simulink model "MIMOSystemAntenna"  (R2021a)
settings: Solver=FixedStepDiscrete  StartTime=0.0  StopTime=inf  RelTol=1e-3
PreLoadFcn:
  | Sig_Ang=120;
  | Int_Ang=90;
  | Frame = 32;
  | load dipoleArray;
InitFcn:
  | load dipoleArray;
values from neighbouring files (symbols this model uses):
  F0 = 5000000000    [dipoleArray.mat]
  L = [9.00164081673e-10 1.08900441217e-09 1.17350873052e-09 1.12597709024e-09 1.12597709023e-09 1.17350873052e-09 1.08900441217e-09 9.00164081661e-10]    [dipoleArray.mat]
  lambda = 0.0599584916    [dipoleArray.mat]
undefined symbols (not defined in the file or in its folder): comm, constellation, design, dipole, if_filt, magnitude, pattern, phased, physconst, rf_filt, S
libraries: simrfV2elements x41, simrfV2util1 x17, simulink_extras x16, simrfV2systems x8, simrfV2sources1 x8, commfilt2 x2, dspmathops x2, commrflib2 x1, dspsrcs4 x1, phasedbflib x1, phaseddoalib x1, commrfcorlib x1
settings Model: SimulationMode=accelerator  NumberOfSteps=8  Creator=shmueld  LastModifiedBy=Michael
settings SolverCC: AlgebraicLoopSolver=TrustRegion  MinimalZcImpactIntegration=on
settings DataIOCC: SaveFormat=Array  SaveOutput=off  SignalLogging=off  DSMLogging=off  VisualizeSimOutput=off  SaveTime=off  ReturnWorkspaceOutputs=off
settings OptimizationCC: DefaultParameterBehavior=Inlined  InlineInvariantSignals=on  EfficientMapNaN2IntZero=off  LifeSpan=inf
settings DebuggingCC: RTPrefix=none  ReadBeforeWriteMsg=DisableAll  WriteAfterWriteMsg=DisableAll  WriteAfterReadMsg=DisableAll  AlgebraicLoopMsg=none  ArtificialAlgebraicLoopMsg=none  MaxConsecutiveZCsMsg=none  InheritedTsInSrcMsg=none  MultiTaskDSMMsg=none  MultiTaskCondExecSysMsg=none  MultiTaskRateTransMsg=warning  TasksWithSamePriorityMsg=none  SigSpecEnsureSampleTimeMsg=none  IntegerOverflowMsg=none  Int32ToFloatConvMsg=none  ParameterDowncastMsg=none  ParameterOverflowMsg=none  ParameterPrecisionLossMsg=none  ParameterTunabilityLossMsg=none  FcnCallInpInsideContextMsg=warning  UnconnectedInputMsg=none  UnconnectedOutputMsg=none  UnconnectedLineMsg=none  FrameProcessingCompatibilityMsg=none  BusObjectLabelMismatch=none  RootOutportRequireBusObject=none  AllowSymbolicDim=off  UnknownTsInhSupMsg=none  ModelReferenceDataLoggingMessage=none  ModelReferenceExtraNoncontSigs=none  OperatingPointInterfaceChecksumMismatchMsg=none  NonCurrentReleaseOperatingPointMsg=warning  PregeneratedLibrarySubsystemCodeDiagnostic=none  SFUnusedDataAndEventsDiag=none  SFUnexpectedBacktrackingDiag=none  SFInvalidInputDataAccessInChartInitDiag=none  SFNoUnconditionalDefaultTransitionDiag=none  SFTransitionOutsideNaturalParentDiag=none  SFUnreachableExecutionPathDiag=none  SFUndirectedBroadcastEventsDiag=none  SFTransitionActionBeforeConditionDiag=none  SFOutputUsedAsStateInMooreChartDiag=none  SFExecutionAtInitializationDiag=none  SFMachineParentedDataDiag=warning  IntegerSaturationMsg=none  ArithmeticOperatorsInVariantConditions=warning
settings HardwareCC: ProdBitPerPointer=32  ProdBitPerSizeT=32  ProdBitPerPtrDiffT=32  ProdLargestAtomicFloat=None  ProdIntDivRoundTo=Undefined  ProdEndianess=Unspecified  ProdWordSize=32  ProdHWDeviceType=32-bit Generic  TargetBitPerPointer=64  TargetBitPerSizeT=64  TargetBitPerPtrDiffT=64  TargetLongLongMode=on  TargetIntDivRoundTo=Zero  TargetEndianess=LittleEndian  TargetWordSize=64  TargetHWDeviceType=MATLAB Host  ProdEqTarget=off
settings ModelReferenceCC: UpdateModelReferenceTargets=IfOutOfDate  PropagateSignalLabelsOutOfModel=off
settings SFSimCC: SFSimEcho=off  SimUseLocalCustomCode=off  CustomCodeUndefinedFunction=UseInterfaceOnly
settings RTWCC: RTWUseLocalCustomCode=off
settings CodeAppCC: MaxIdLength=128
settings GRTTargetCC: TargetLangStandard=C89/C90 (ANSI)  CombineOutputUpdateFcns=off  GRTInterface=on
settings ConfigComp: CovMetricSettings=dw  CovSaveCumulativeToWorkspaceVar=on  CovSaveSingleToWorkspaceVar=on  CovExternalEMLEnable=off
settings SimscapeCC: ExplicitSolverDiagnosticOptions=none  SimscapeNormalizeSystem=off

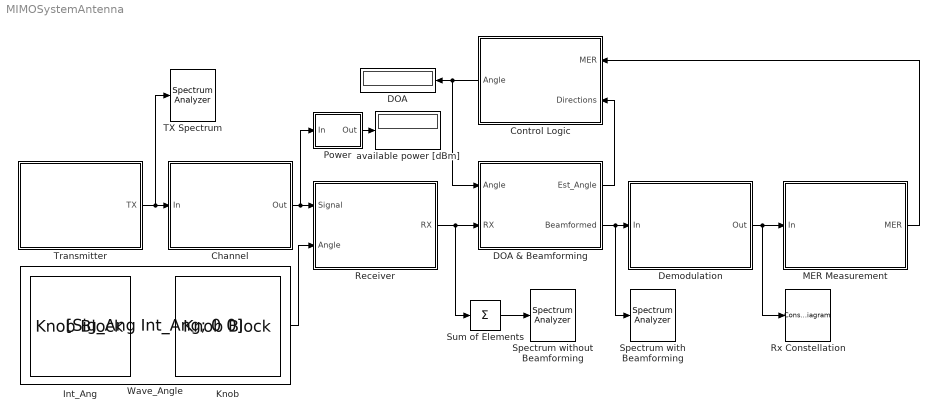
== system MIMOSystemAntenna ==
  Channel : Subsystem  mask{PathLoss=60, PowInterf=-20}
      mask prompts: PathLoss "Path loss (dB)"; PowInterf "Interfering signal power (dBm)"
  Control Logic : Subsystem
  DOA : Display
  DOA & Beamforming : Subsystem
  Demodulation : Subsystem
  Int_Ang : KnobBlock  ScaleMax=180  TickInterval=30
  Knob : KnobBlock  ScaleMax=180  TickInterval=30
  MER Measurement : Subsystem
  "Power  " : Subsystem  mask{R=1}
      mask prompts: R "Reference Impedance [Ohm]"
      mask DialogControl DescGroupVar Prompt: Power Meter
  Receiver : Subsystem
  Rx Constellation : ConstellationDiagram
  Spectrum with Beamforming : SpectrumAnalyzer
  Spectrum without Beamforming : SpectrumAnalyzer
  Sum of Elements : Sum  Inputs=+
  TX Spectrum : SpectrumAnalyzer
  Transmitter : Subsystem
  Wave_Angle : Constant  Value=[Sig_Ang Int_Ang; 0 0]  VectorParams1D=off
      mask Display: disp('')
  available power [dBm] : Display
  wires:
  DOA & Beamforming/2(Beamformed) -> Demodulation/1(In), Spectrum with Beamforming/1
  Sum of Elements/1 -> Spectrum without Beamforming/1
  Transmitter/1(TX) -> TX Spectrum/1, Channel/1(In)
  Receiver/1(RX) -> Sum of Elements/1, DOA & Beamforming/2(RX)
  Channel/1(Out) -> "Power  "/1(In), Receiver/1(Signal)
  Wave_Angle/1 -> Receiver/2(Angle)
  Control Logic/1(Angle) -> DOA & Beamforming/1(Angle), DOA/1
  MER Measurement/1(MER) -> Control Logic/1(MER)
  DOA & Beamforming/1(Est_Angle) -> Control Logic/2(Directions)
  Demodulation/1(Out) -> MER Measurement/1(In), Rx Constellation/1
  "Power  "/1(Out) -> available power [dBm]/1

== system MIMOSystemAntenna/Channel ==
  In : Inport
  Free Space Path Loss1 : commrflib2/Free Space Path Loss  mode=Decibels  dB=PathLoss  d=0.100  fc=1920
      settings: SourceProductBaseCode=CM
  Interferer : dspsrcs4/Sine Wave  Amplitude=10^((PowInterf-30)/20)  Frequency=2.5e6  Phase=0  SampleMode=Discrete  OutComplex=Complex  CompMethod=Trigonometric fcn  TableSize=Speed  SampleTime=8.6806e-8  SamplesPerFrame=1  ResetState=Restart at time zero  OutputFrames=off  dataType=double  wordLen=16  udDataType=sfix(16)  fracBitsMode=Best precision  numFracBits=15  OutDataTypeStr=double  LastOutDataTypeStr=double
  Vector Concatenate1 : Concatenate  Mode=Multidimensional array  ConcatenateDimension=2
  Out : Outport  VectorParamsAs1DForOutWhenUnconnected=off
  wires:
  Free Space Path Loss1/1 -> Vector Concatenate1/1  "Input RX"
  Vector Concatenate1/1 -> Out/1
  In/1 -> Free Space Path Loss1/1
  Interferer/1 -> Vector Concatenate1/2

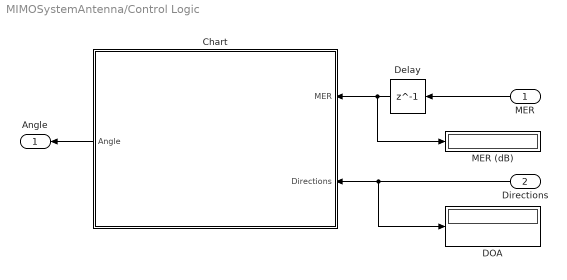
== system MIMOSystemAntenna/Control Logic ==
  MER : Inport
  Directions : Inport  Port=2
  Chart : Stateflow chart  TreatAsAtomicUnit=on
  DOA : Display
  Delay : Delay  DelayLength=1  InitialCondition=0
  MER (dB) : Display
  Angle : Outport  VectorParamsAs1DForOutWhenUnconnected=off
  wires:
  Delay/1 -> Chart/1(MER), MER (dB)/1
  Directions/1 -> Chart/2(Directions), DOA/1
  Chart/1(Angle) -> Angle/1
  MER/1 -> Delay/1

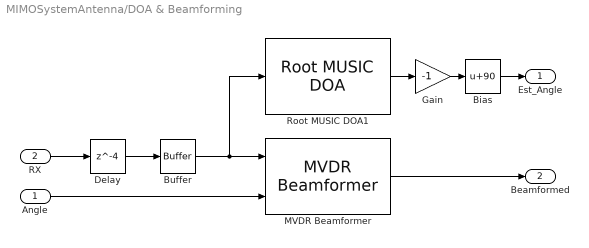
== system MIMOSystemAntenna/DOA & Beamforming ==
  Angle : Inport
  RX : Inport  Port=2
  Bias : Bias  Bias=90
  Buffer : Buffer  N=Frame  OutputFrames=off
  Delay : Delay  DelayLength=4  InitialCondition=1
  Gain : Gain  Gain=-1
  MVDR Beamformer : phasedbflib/MVDR Beamformer  PropagationSpeed=physconst( 'LightSpeed' )  OperatingFrequency=F0  DiagonalLoadingFactor=0.1  TrainingInputPort=off  DirectionSource=Input port  Direction=[ 0; 0 ]  NumPhaseShifterBits=0  WeightsOutputPort=off  SimulateUsing=Interpreted execution  SensorArray=phased.ULA('Element',phased.CustomAntennaElement('AzimuthAngles',-180:5:180,'ElevationAngles',-90:5:90,'MagnitudePattern',pattern(design(dipole,F0), F0),'PhasePattern',zeros(37,73)),'NumElements',8,'ElementSpacing',0.5*lambda,'ArrayAxis','x')
      settings: SourceProductBaseCode=AR
  Root MUSIC DOA1 : phaseddoalib/Root MUSIC DOA  PropagationSpeed=physconst( 'LightSpeed' )  OperatingFrequency=F0  NumSignalsSource=Property  NumSignalsMethod=AIC  NumSignals=2  ForwardBackwardAveraging=on  SpatialSmoothing=0  SimulateUsing=Interpreted execution  SensorArray=phased.ULA('Element',phased.CustomAntennaElement('AzimuthAngles',-180:5:180,'ElevationAngles',-90:5:90,'MagnitudePattern',pattern(design(dipole,F0), F0),'PhasePattern',zeros(37,73)),'NumElements',8,'ArrayAxis','x','ElementSpacing',0.5*lambda)
      settings: SourceProductBaseCode=AR
  Est_Angle : Outport  VectorParamsAs1DForOutWhenUnconnected=off
  Beamformed : Outport  Port=2  VectorParamsAs1DForOutWhenUnconnected=off
  wires:
  Gain/1 -> Bias/1
  Bias/1 -> Est_Angle/1
  RX/1 -> Delay/1
  Root MUSIC DOA1/1 -> Gain/1
  Buffer/1 -> MVDR Beamformer/1, Root MUSIC DOA1/1
  MVDR Beamformer/1 -> Beamformed/1
  Delay/1 -> Buffer/1
  Angle/1 -> MVDR Beamformer/2

== system MIMOSystemAntenna/Demodulation ==
  In : Inport
  AGC : commrfcorlib/AGC  LegacyMode=off  DetectorMethod=Rectifier  LoopMethod=Linear  UpdatePeriod=100  StepSize=0.1  AdaptationStepSize=0.01  DesiredOutputPower=1/8  AveragingLength=64  MaximumGain=30  MaxPowerGain=60  GainOutputPort=off  InputPowerOutputPort=off  SimulateUsing=Interpreted execution
  Raised Cosine Receive Filter : commfilt2/Raised Cosine Receive Filter  filtType=Square root  R=0.2  filtSpan=8  N=8  downFactor=8  downOffset=0  filterGain=1  InputProcessing=Columns as channels (frame based)  RateOptions=Enforce single-rate processing  framing=Mute  checkCoeff=off  variableName=rcRxFilt  currentFiltSpan=8  D=(8)/2  inputOffset=0  sampMode=Mute  saveAsFlag=0  rateMode=Downsampling  checkGain=Normalized  launchFVT=on  roundingMode=Floor  overflowMode=off  coeffDataTypeStr=Inherit: Same word length as input  coeffMin=[]  coeffMax=[]  coeffLastDataTypeStr=Inherit: Same word length as input  accumDataTypeStr=Inherit: Same as product output  accumLastDataTypeStr=Inherit: Same as product output  outputDataTypeStr=Inherit: Same as accumulator  outputMin=[]  outputMax=[]  outputLastDataTypeStr=Inherit: Same as accumulator
  Out : Outport  VectorParamsAs1DForOutWhenUnconnected=off
      settings: SignalType=complex
  wires:
  AGC/1 -> Raised Cosine Receive Filter/1
  In/1 -> AGC/1
  Raised Cosine Receive Filter/1 -> Out/1

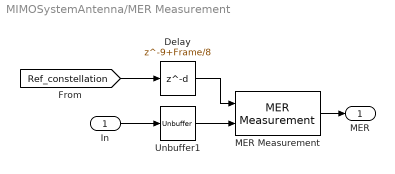
== system MIMOSystemAntenna/MER Measurement ==
  In : Inport
  Delay : Delay  DelayLength=9+Frame/8
  MER Measurement : commutil2/MER Measurement  ReferenceSignalSource=Input port  ReferenceConstellation=constellation( comm.QPSKModulator )  MeasurementIntervalSource=Custom  MeasurementInterval=8  AveragingDimensions=1  MinimumMEROutputPort=off  XPercentileMEROutputPort=off  XPercentileValue=95  SymbolCountOutputPort=off  SimulateUsing=Interpreted execution
      settings: SourceProductBaseCode=CM
  Unbuffer1 : Unbuffer
  MER : Outport  VectorParamsAs1DForOutWhenUnconnected=off
  wires:
  MER Measurement/1 -> MER/1
  Delay/1 -> MER Measurement/1
  [Ref_constellation] -> Delay/1
  In/1 -> Unbuffer1/1
  Unbuffer1/1 -> MER Measurement/2

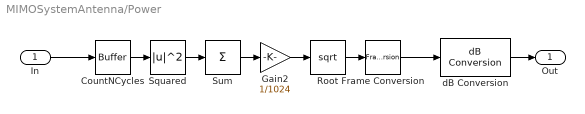
== system MIMOSystemAntenna/Power   ==
  In : Inport
  CountNCycles : Buffer  N=1024
  Frame Conversion : FrameConversion  OutFrame=Sample-based
  Gain2 : Gain  Gain=1/1024
  Root : Sqrt  SaturateOnIntegerOverflow=on
  Squared : Math  Operator=magnitude^2  SignedPower=on  SaturateOnIntegerOverflow=on
  Sum : Sum  Inputs=+  CollapseMode=Specified dimension
  dB Conversion : dspmathops/dB Conversion  dBtype=dBm  intype=Amplitude  R=R  fuzz=on
  Out : Outport  VectorParamsAs1DForOutWhenUnconnected=off
  wires:
  dB Conversion/1 -> Out/1
  In/1 -> CountNCycles/1
  Frame Conversion/1 -> dB Conversion/1
  CountNCycles/1 -> Squared/1
  Squared/1 -> Sum/1
  Sum/1 -> Gain2/1
  Root/1 -> Frame Conversion/1
  Gain2/1 -> Root/1

== system MIMOSystemAntenna/Receiver ==
  Signal : Inport
  Angle : Inport  Port=2
  Narrowband_Receive_Array : phasedtxrxlib/Narrowband Receive Array  PropagationSpeed=physconst( 'LightSpeed' )  OperatingFrequency=F0  Wavefront=Plane  SensorGainMeasure=dB  Polarization=None  WeightsInputPort=off  SimulateUsing=Interpreted execution  Sensor=phased.ULA('Element',phased.CustomAntennaElement('AzimuthAngles',-180:5:180,'ElevationAngles',-90:5:90,'MagnitudePattern',pattern(design(dipole,F0), F0),'PhasePattern',zeros(37,73)),'NumElements',8,'ElementSpacing',0.5*lambda,'ArrayAxis','x')
      settings: SourceProductBaseCode=AR
  RF_Receiver : Subsystem
  RX : Outport  VectorParamsAs1DForOutWhenUnconnected=off
  wires:
  Angle/1 -> Narrowband_Receive_Array/2
  Signal/1 -> Narrowband_Receive_Array/1
  Narrowband_Receive_Array/1 -> RF_Receiver/1(In)
  RF_Receiver/1(Out) -> RX/1

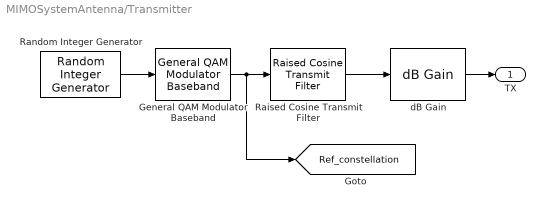
== system MIMOSystemAntenna/Transmitter ==
  General QAM Modulator Baseband : commdigbbndam3/General QAM Modulator Baseband  SigCon=[exp(2*pi*1i*[0:7]/8)]  outDtype=double  outWordLen=16  outUDDataType=sfix(16)  outFracLenMode=Best precision  outFracLen=15  outDataTypeStr=double  outLastDataTypeStr=double
      settings: SourceProductBaseCode=CM
  Raised Cosine Transmit Filter : commfilt2/Raised Cosine Transmit Filter  filtType=Square root  R=0.2  filtSpan=8  N=8  filterGain=1  InputProcessing=Columns as channels (frame based)  RateOptions=Allow multirate processing  framing=Mute  checkCoeff=off  variableName=rcTxFilt  checkGain=Normalized  sampMode=Mute  saveAsFlag=0  currentFiltSpan=8  D=(8)/2  launchFVT=on  roundingMode=Floor  overflowMode=off  coeffDataTypeStr=Inherit: Same word length as input  coeffMin=[]  coeffMax=[]  coeffLastDataTypeStr=Inherit: Same word length as input  outputDataTypeStr=Inherit: Same as accumulator  outputMin=[]  outputMax=[]  outputLastDataTypeStr=Inherit: Same as accumulator
  Random Integer Generator : commrandsrc3/Random Integer Generator  SetSize=8  SeedSource=Parameter  Seed=123456  SampleTime=8.6806e-8*8  SamplesPerFrame=1  OutputDataType=double  SimulateUsing=Interpreted execution
  dB Gain : dspmathops/dB Gain  dB=20  intype=Amplitude
      settings: SourceProductBaseCode=DS
  TX : Outport  VectorParamsAs1DForOutWhenUnconnected=off
  tag scope: Ref_constellation=global
  wires:
  Raised Cosine Transmit Filter/1 -> dB Gain/1
  General QAM Modulator Baseband/1 -> [Ref_constellation], Raised Cosine Transmit Filter/1
  Random Integer Generator/1 -> General QAM Modulator Baseband/1
  dB Gain/1 -> TX/1

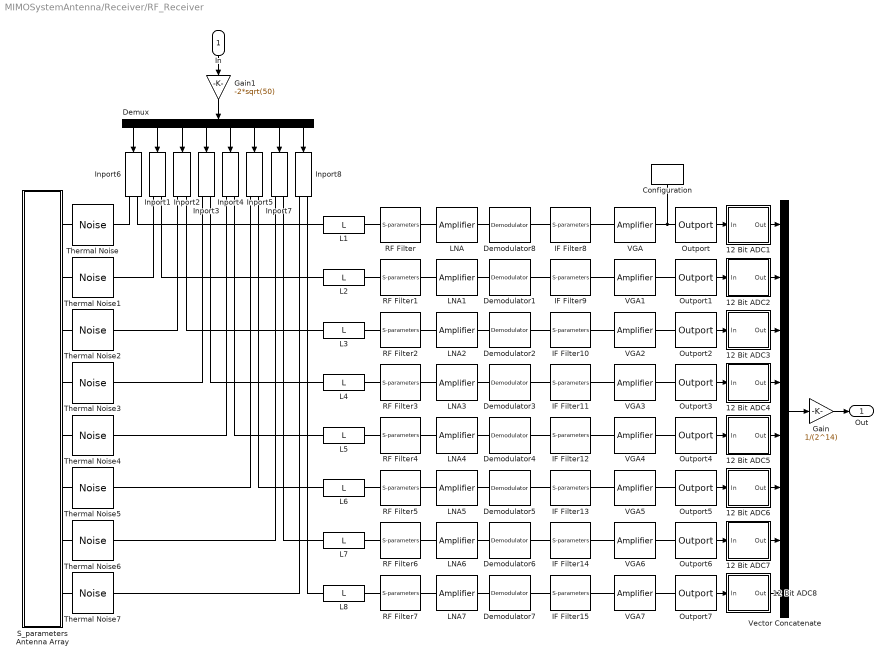
== system MIMOSystemAntenna/Receiver/RF_Receiver ==
  In : Inport
  12 Bit ADC1 : Subsystem  mask{FS_P_dBm=18, N=12}
      mask prompts: FS_P_dBm "Full Scale Power (dBm)"
  12 Bit ADC2 : Subsystem  mask{FS_P_dBm=18, N=12}
      mask prompts: FS_P_dBm "Full Scale Power (dBm)"
  12 Bit ADC3 : Subsystem  mask{FS_P_dBm=18, N=12}
      mask prompts: FS_P_dBm "Full Scale Power (dBm)"
  12 Bit ADC4 : Subsystem  mask{FS_P_dBm=18, N=12}
      mask prompts: FS_P_dBm "Full Scale Power (dBm)"
  12 Bit ADC5 : Subsystem  mask{FS_P_dBm=18, N=12}
      mask prompts: FS_P_dBm "Full Scale Power (dBm)"
  12 Bit ADC6 : Subsystem  mask{FS_P_dBm=18, N=12}
      mask prompts: FS_P_dBm "Full Scale Power (dBm)"
  12 Bit ADC7 : Subsystem  mask{FS_P_dBm=18, N=12}
      mask prompts: FS_P_dBm "Full Scale Power (dBm)"
  12 Bit ADC8 : Subsystem  mask{FS_P_dBm=18, N=12}
      mask prompts: FS_P_dBm "Full Scale Power (dBm)"
  Configuration : simrfV2util1/Configuration  AutoFreq=off  Tones=[0.07 5] GHz  Harmonics=[1 3]  NormalizeCarrierPower=on  SolverType=Auto  UseCCode=on  StepSize=8.6806e-8 s  AddNoise=off  defaultRNG=on  Seed=0  Temperature=290.0 K  SolverDelFlag=0  AbsTol=1e-6  RelTol=1e-3  MaxIter=10  ErrorEstimationType=2-norm over all variables  EnableInterpFilter=off  HiddenFIRfilterControllerParam=off  SmallSignalApprox=off  AllSimFreqs=on  SimFreqs=[] Hz  SimFreqsInternal=[]  SamplesPerFrame=1
      settings: SourceProductBaseCode=RB
  Demodulator{1..8} (8 alike) : simrfV2systems/Demodulator  classname=rfdemod  Source_linear_gain=Available power gain  linear_gain=-6 dB  Poly_Coeffs=[0 1]  LOFreq=4.93 GHz  Zin=50  Zout=50  AddIRFilter=on  AddCSFilter=on  InternalGrounding=on  ForceNextInit=off  Source_Poly=Even and odd order  IPType=Input  IP2=inf dBm  IP3=32 dBm  P1dB=inf dBm  Psat=inf dBm  Gcomp=inf dBm  NF=5.4  Isolation=inf dB  AddPhaseNoise=on  PhaseNoiseOffset=[1e5 2e5 1e6]  PhaseNoiseLevel=[-90 -100 -140]  AutoImpulseLengthPN=on  ImpulseLengthPN=1e-10  ImpulseLength_unitPN=s  DesignMethodIR=Ideal  ResponseTypeIR=Highpass  ImplementationIR=LC Tee  ImplementationIdealIR=Constant per carrier  ImplementationRationalIR=Transfer function  UseFilterOrderIR=on  FilterOrderIR=3  PassFreq_lpIR=1  PassFreq_lp_unitIR=GHz  PassFreq_hpIR=2  PassFreq_hp_unitIR=GHz  PassFreq_bpIR=[2 3]  PassFreq_bp_unitIR=GHz  PassFreq_bsIR=[1 4]  PassFreq_bs_unitIR=GHz  PassAttenIR=10*log10(2)  StopFreq_lpIR=2  StopFreq_lp_unitIR=GHz  StopFreq_hpIR=1  StopFreq_hp_unitIR=GHz  StopFreq_bpIR=[1.5 3.5]  StopFreq_bp_unitIR=GHz  StopFreq_bsIR=[2.1 2.9]  StopFreq_bs_unitIR=GHz  StopAttenIR=40  RsrcIR=50  RloadIR=50  AutoImpulseLengthIR=on  ImpulseLengthIR=1e-10  ImpulseLength_unitIR=s  DesignMethodCS=Ideal  ResponseTypeCS=Lowpass  ImplementationCS=LC Tee  ImplementationIdealCS=Constant per carrier  ImplementationRationalCS=Transfer function  UseFilterOrderCS=on  FilterOrderCS=3  PassFreq_lpCS=1  PassFreq_lp_unitCS=GHz  PassFreq_hpCS=2  PassFreq_hp_unitCS=GHz  PassFreq_bpCS=[2 3]  PassFreq_bp_unitCS=GHz  PassFreq_bsCS=[1 4]  PassFreq_bs_unitCS=GHz  PassAttenCS=10*log10(2)  StopFreq_lpCS=2  StopFreq_lp_unitCS=GHz  StopFreq_hpCS=1  StopFreq_hp_unitCS=GHz  StopFreq_bpCS=[1.5 3.5]  StopFreq_bp_unitCS=GHz  StopFreq_bsCS=[2.1 2.9]  StopFreq_bs_unitCS=GHz  StopAttenCS=40  RsrcCS=50  RloadCS=50  AutoImpulseLengthCS=on  ImpulseLengthCS=1e-10  ImpulseLength_unitCS=s
      settings: SourceProductBaseCode=RB
  Demux : Demux  Outputs=8
  Gain : Gain  Gain=1/(2^14)
  Gain1 : Gain  Gain=-2*sqrt(50)
  IF Filter{8..15} (8 alike) : simrfV2elements/S-parameters  classname=sparam_element  DataSource=Data file  File=.\if_filt.s2p  Paramtype=S-parameters  Sparam=[0 0;1 0]  SparamFreq=1e9 Hz  SparamZ0=50  Residues=0  Poles=0  DF={0 0; 1 0}  FitOpt=Share all poles  FitTol=-20  SourceFreq=Extracted from data source  PlotFreq=[1e9:1e6:3e9] Hz  PlotType=X-Y plane  YParam1=S(2,1)  YFormat1=Magnitude (decibels)  YParam2=None  YFormat2=Magnitude (decibels)  YOption=Linear  XOption=Linear  AddNoise=off  InternalGrounding=on  SparamRepresentation=Frequency domain  AutoImpulseLength=on  ImpulseLength=256*8.6806e-8 s  MagModeling=off  CacheLevel=0
      settings: SourceProductBaseCode=RB
  Inport{1..8} (8 alike) : simrfV2util1/Inport  SimulinkInputSignalType=Ideal voltage  CarrierFreq=F0 Hz  ZS=0  InternalGrounding=off
      settings: SourceProductBaseCode=RB
  L1 : simrfV2elements/L  classname=inductor  Inductance=L(1) H
      settings: SourceProductBaseCode=RB
  L2 : simrfV2elements/L  classname=inductor  Inductance=L(2) H
      settings: SourceProductBaseCode=RB
  L3 : simrfV2elements/L  classname=inductor  Inductance=L(3) H
      settings: SourceProductBaseCode=RB
  L4 : simrfV2elements/L  classname=inductor  Inductance=L(4) H
      settings: SourceProductBaseCode=RB
  L5 : simrfV2elements/L  classname=inductor  Inductance=L(5) H
      settings: SourceProductBaseCode=RB
  L6 : simrfV2elements/L  classname=inductor  Inductance=L(6) H
      settings: SourceProductBaseCode=RB
  L7 : simrfV2elements/L  classname=inductor  Inductance=L(7) H
      settings: SourceProductBaseCode=RB
  L8 : simrfV2elements/L  classname=inductor  Inductance=L(8) H
      settings: SourceProductBaseCode=RB
  LNA{,1..7} (8 alike) : simrfV2elements/Amplifier  classname=amplifier  DataSource=Data file  File=unitygain.s2p  Paramtype=S-parameters  Sparam=[0 0;1 0]  SparamFreq=1e9 Hz  SparamZ0=50  Residues=0  Poles=0  DF={0 0; 1 0}  Source_linear_gain=Available power gain  linear_gain=12 dB  Zin=50  Zout=50  Source_Poly=Even and odd order  Poly_Coeffs=[0 1]  IPType=Output  IP2=Inf dBm  IP3=21 dBm  P1dB=inf dBm  Psat=inf dBm  Gcomp=inf dBm  InternalGrounding=on  SourceFreq=Extracted from data source  PlotFreq=[1e9:1e6:3e9] Hz  PlotType=X-Y plane  YParam1=S(1,1)  YFormat1=Magnitude (decibels)  YParam2=None  YFormat2=Magnitude (decibels)  YOption=Linear  XOption=Linear  SparamRepresentation=Time domain (rationalfit)  FitTol=-40  FitOpt=Fit individually  AutoImpulseLength=on  ImpulseLength=1e-10 s  MagModeling=off  AddNoise=on  NoiseType=Noise figure  NoiseDist=White  NF=1.3  MinNF=0  Gopt=0  RN=0  CarrierFreq=0 Hz  NoiseAutoImpulseLength=on  NoiseImpulseLength=1e-10 s  SpecifyOpFreq=off  OpFreq=0 Hz
      settings: SourceProductBaseCode=RB
  Outport{,1..7} (8 alike) : simrfV2util1/Outport  SensorType=Power  OutputFormat=Complex Baseband  CarrierFreq=70 MHz  ZL=50  InternalGrounding=on  StepSize=1e-6 s  AutoStep=on
      settings: SourceProductBaseCode=RB
  RF Filter{,1..7} (8 alike) : simrfV2elements/S-parameters  classname=sparam_element  DataSource=Data file  File=.\rf_filt.s2p  Paramtype=S-parameters  Sparam=[0 0;1 0]  SparamFreq=1e9 Hz  SparamZ0=50  Residues=0  Poles=0  DF={0 0; 1 0}  FitOpt=Share all poles  FitTol=-20  SourceFreq=Extracted from data source  PlotFreq=[1e9:1e6:3e9] Hz  PlotType=X-Y plane  YParam1=S(2,1)  YFormat1=Magnitude (decibels)  YParam2=None  YFormat2=Magnitude (decibels)  YOption=Linear  XOption=Linear  AddNoise=off  InternalGrounding=on  SparamRepresentation=Frequency domain  AutoImpulseLength=on  ImpulseLength=1e-10 s  MagModeling=off  CacheLevel=0
      settings: SourceProductBaseCode=RB
  S_parameters Antenna Array : Subsystem
  Thermal Noise{,1..7} (8 alike) : simrfV2sources1/Noise  SimulinkInputSignalType=Ideal voltage  NoiseType=White  NoisePSD=4*physconst('Boltzmann')*290*50  CarrierFreq=0 Hz  AutoImpulseLength=on  ImpulseLength=1e-10 s  InternalGrounding=off
      settings: SourceProductBaseCode=RB
  VGA{,1..7} (8 alike) : simrfV2elements/Amplifier  classname=amplifier  DataSource=Data file  File=unitygain.s2p  Paramtype=S-parameters  Sparam=[0 0;1 0]  SparamFreq=1e9 Hz  SparamZ0=50  Residues=0  Poles=0  DF={0 0; 1 0}  Source_linear_gain=Available power gain  linear_gain=20 dB  Zin=50  Zout=50  Source_Poly=Even and odd order  Poly_Coeffs=[0 1]  IPType=Output  IP2=Inf dBm  IP3=Inf dBm  P1dB=inf dBm  Psat=inf dBm  Gcomp=inf dBm  InternalGrounding=on  SourceFreq=Extracted from data source  PlotFreq=[1e9:1e6:3e9] Hz  PlotType=X-Y plane  YParam1=S(1,1)  YFormat1=Magnitude (decibels)  YParam2=None  YFormat2=Magnitude (decibels)  YOption=Linear  XOption=Linear  SparamRepresentation=Time domain (rationalfit)  FitTol=-40  FitOpt=Fit individually  AutoImpulseLength=on  ImpulseLength=1e-10 s  MagModeling=off  AddNoise=on  NoiseType=Noise figure  NoiseDist=White  NF=6  MinNF=0  Gopt=0  RN=0  CarrierFreq=0 Hz  NoiseAutoImpulseLength=on  NoiseImpulseLength=1e-10 s  SpecifyOpFreq=off  OpFreq=0 Hz
      settings: SourceProductBaseCode=RB
  Vector Concatenate : Concatenate  NumInputs=8  Mode=Multidimensional array  ConcatenateDimension=2
  Out : Outport  VectorParamsAs1DForOutWhenUnconnected=off
  wires:
  In/1 -> Gain1/1
  12 Bit ADC1/1(Out) -> Vector Concatenate/1
  12 Bit ADC2/1(Out) -> Vector Concatenate/2
  12 Bit ADC4/1(Out) -> Vector Concatenate/4
  12 Bit ADC5/1(Out) -> Vector Concatenate/5
  12 Bit ADC6/1(Out) -> Vector Concatenate/6
  12 Bit ADC7/1(Out) -> Vector Concatenate/7
  Gain1/1 -> Demux/1
  Demux/2 -> Inport1/1
  Demux/3 -> Inport2/1
  Demux/4 -> Inport3/1
  Demux/5 -> Inport4/1
  Demux/6 -> Inport5/1
  Demux/7 -> Inport7/1
  Demux/8 -> Inport8/1
  Demux/1 -> Inport6/1
  Outport6/1 -> 12 Bit ADC7/1("In  ")
  Outport5/1 -> 12 Bit ADC6/1("In  ")
  Outport4/1 -> 12 Bit ADC5/1("In  ")
  Outport3/1 -> 12 Bit ADC4/1("In  ")
  Outport2/1 -> 12 Bit ADC3/1("In  ")
  Outport1/1 -> 12 Bit ADC2/1("In  ")
  Vector Concatenate/1 -> Gain/1
  Outport/1 -> 12 Bit ADC1/1("In  ")
  12 Bit ADC3/1(Out) -> Vector Concatenate/3
  12 Bit ADC8/1(Out) -> Vector Concatenate/8
  Outport7/1 -> 12 Bit ADC8/1("In  ")
  Gain/1 -> Out/1
  connections:
  Thermal Noise/RConn1 -- S_parameters Antenna Array/RConn1
  Thermal Noise1/RConn1 -- S_parameters Antenna Array/RConn2
  Thermal Noise2/RConn1 -- S_parameters Antenna Array/RConn3
  Thermal Noise3/RConn1 -- S_parameters Antenna Array/RConn4
  Thermal Noise4/RConn1 -- S_parameters Antenna Array/RConn5
  Thermal Noise5/LConn1 -- Inport5/RConn1
  Thermal Noise6/LConn1 -- Inport7/RConn1
  Thermal Noise7/LConn1 -- Inport8/RConn1
  Configuration/LConn1 -- Outport/LConn1 -- VGA/RConn1
  Inport2/RConn2 -- L3/LConn1
  Inport5/RConn2 -- L6/LConn1
  Inport8/RConn2 -- L8/LConn1
  Inport1/RConn2 -- L2/LConn1
  Thermal Noise4/LConn1 -- Inport4/RConn1
  Thermal Noise3/LConn1 -- Inport3/RConn1
  Thermal Noise7/RConn1 -- S_parameters Antenna Array/RConn8
  Thermal Noise2/LConn1 -- Inport2/RConn1
  Thermal Noise/LConn1 -- Inport6/RConn1
  Thermal Noise1/LConn1 -- Inport1/RConn1
  Thermal Noise5/RConn1 -- S_parameters Antenna Array/RConn6
  Thermal Noise6/RConn1 -- S_parameters Antenna Array/RConn7
  Inport4/RConn2 -- L5/LConn1
  Inport3/RConn2 -- L4/LConn1
  Inport6/RConn2 -- L1/LConn1
  Inport7/RConn2 -- L7/LConn1
  VGA1/RConn1 -- Outport1/LConn1
  IF Filter10/RConn1 -- VGA2/LConn1
  VGA3/RConn1 -- Outport3/LConn1
  IF Filter12/RConn1 -- VGA4/LConn1
  IF Filter13/RConn1 -- VGA5/LConn1
  VGA6/RConn1 -- Outport6/LConn1
  VGA7/RConn1 -- Outport7/LConn1
  LNA/RConn1 -- Demodulator8/LConn1
  RF Filter1/LConn1 -- L2/RConn1
  RF Filter2/LConn1 -- L3/RConn1
  RF Filter3/LConn1 -- L4/RConn1
  RF Filter4/LConn1 -- L5/RConn1
  RF Filter5/LConn1 -- L6/RConn1
  RF Filter6/LConn1 -- L7/RConn1
  RF Filter7/LConn1 -- L8/RConn1
  IF Filter8/LConn1 -- Demodulator8/RConn1
  IF Filter9/LConn1 -- Demodulator1/RConn1
  IF Filter10/LConn1 -- Demodulator2/RConn1
  IF Filter11/LConn1 -- Demodulator3/RConn1
  IF Filter12/LConn1 -- Demodulator4/RConn1
  IF Filter13/LConn1 -- Demodulator5/RConn1
  IF Filter14/LConn1 -- Demodulator6/RConn1
  IF Filter15/LConn1 -- Demodulator7/RConn1
  IF Filter9/RConn1 -- VGA1/LConn1
  IF Filter8/RConn1 -- VGA/LConn1
  IF Filter15/RConn1 -- VGA7/LConn1
  VGA5/RConn1 -- Outport5/LConn1
  IF Filter14/RConn1 -- VGA6/LConn1
  VGA4/RConn1 -- Outport4/LConn1
  IF Filter11/RConn1 -- VGA3/LConn1
  VGA2/RConn1 -- Outport2/LConn1
  LNA6/RConn1 -- Demodulator6/LConn1
  LNA2/RConn1 -- Demodulator2/LConn1
  L1/RConn1 -- RF Filter/LConn1
  LNA1/RConn1 -- Demodulator1/LConn1
  LNA4/RConn1 -- Demodulator4/LConn1
  LNA5/RConn1 -- Demodulator5/LConn1
  LNA7/RConn1 -- Demodulator7/LConn1
  LNA3/RConn1 -- Demodulator3/LConn1
  RF Filter2/RConn1 -- LNA2/LConn1
  RF Filter6/RConn1 -- LNA6/LConn1
  RF Filter/RConn1 -- LNA/LConn1
  RF Filter1/RConn1 -- LNA1/LConn1
  RF Filter4/RConn1 -- LNA4/LConn1
  RF Filter5/RConn1 -- LNA5/LConn1
  RF Filter7/RConn1 -- LNA7/LConn1
  RF Filter3/RConn1 -- LNA3/LConn1

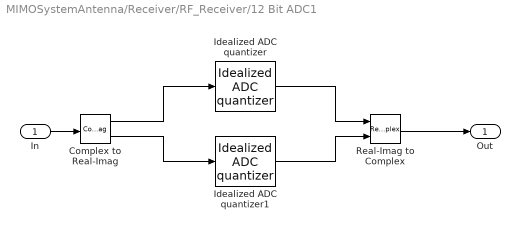
== system MIMOSystemAntenna/Receiver/RF_Receiver/12 Bit ADC1 ==
  "In  " : Inport
  Complex to Real-Imag : ComplexToRealImag
  Idealized ADC quantizer : simulink_extras/Additional Discrete/Idealized ADC quantizer  NumberOfConverterBits=N  Vmin=-10^((FS_P_dBm-30)/20)  Vmax=10^((FS_P_dBm-30)/20)  OutputDataType=double  OutputNegativeValues=on
  Idealized ADC quantizer1 : simulink_extras/Additional Discrete/Idealized ADC quantizer  NumberOfConverterBits=N  Vmin=-10^((FS_P_dBm-30)/20)  Vmax=10^((FS_P_dBm-30)/20)  OutputDataType=double  OutputNegativeValues=on
  Real-Imag to Complex : RealImagToComplex
  Out : Outport  VectorParamsAs1DForOutWhenUnconnected=off
  wires:
  "In  "/1 -> Complex to Real-Imag/1
  Complex to Real-Imag/1 -> Idealized ADC quantizer/1
  Complex to Real-Imag/2 -> Idealized ADC quantizer1/1
  Idealized ADC quantizer/1 -> Real-Imag to Complex/1
  Idealized ADC quantizer1/1 -> Real-Imag to Complex/2
  Real-Imag to Complex/1 -> Out/1

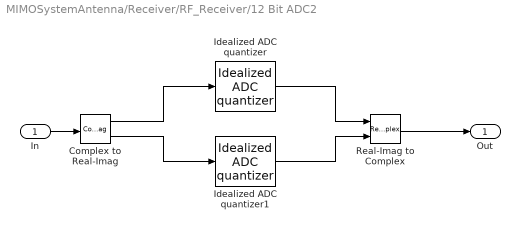
== system MIMOSystemAntenna/Receiver/RF_Receiver/12 Bit ADC2 ==
  "In  " : Inport
  Complex to Real-Imag : ComplexToRealImag
  Idealized ADC quantizer : simulink_extras/Additional Discrete/Idealized ADC quantizer  NumberOfConverterBits=N  Vmin=-10^((FS_P_dBm-30)/20)  Vmax=10^((FS_P_dBm-30)/20)  OutputDataType=double  OutputNegativeValues=on
  Idealized ADC quantizer1 : simulink_extras/Additional Discrete/Idealized ADC quantizer  NumberOfConverterBits=N  Vmin=-10^((FS_P_dBm-30)/20)  Vmax=10^((FS_P_dBm-30)/20)  OutputDataType=double  OutputNegativeValues=on
  Real-Imag to Complex : RealImagToComplex
  Out : Outport  VectorParamsAs1DForOutWhenUnconnected=off
  wires:
  Real-Imag to Complex/1 -> Out/1
  Idealized ADC quantizer1/1 -> Real-Imag to Complex/2
  Idealized ADC quantizer/1 -> Real-Imag to Complex/1
  Complex to Real-Imag/2 -> Idealized ADC quantizer1/1
  Complex to Real-Imag/1 -> Idealized ADC quantizer/1
  "In  "/1 -> Complex to Real-Imag/1

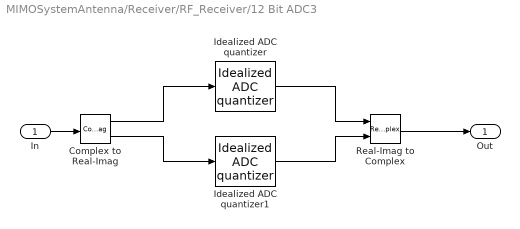
== system MIMOSystemAntenna/Receiver/RF_Receiver/12 Bit ADC3 ==
  "In  " : Inport
  Complex to Real-Imag : ComplexToRealImag
  Idealized ADC quantizer : simulink_extras/Additional Discrete/Idealized ADC quantizer  NumberOfConverterBits=N  Vmin=-10^((FS_P_dBm-30)/20)  Vmax=10^((FS_P_dBm-30)/20)  OutputDataType=double  OutputNegativeValues=on
  Idealized ADC quantizer1 : simulink_extras/Additional Discrete/Idealized ADC quantizer  NumberOfConverterBits=N  Vmin=-10^((FS_P_dBm-30)/20)  Vmax=10^((FS_P_dBm-30)/20)  OutputDataType=double  OutputNegativeValues=on
  Real-Imag to Complex : RealImagToComplex
  Out : Outport  VectorParamsAs1DForOutWhenUnconnected=off
  wires:
  "In  "/1 -> Complex to Real-Imag/1
  Complex to Real-Imag/1 -> Idealized ADC quantizer/1
  Complex to Real-Imag/2 -> Idealized ADC quantizer1/1
  Idealized ADC quantizer/1 -> Real-Imag to Complex/1
  Idealized ADC quantizer1/1 -> Real-Imag to Complex/2
  Real-Imag to Complex/1 -> Out/1

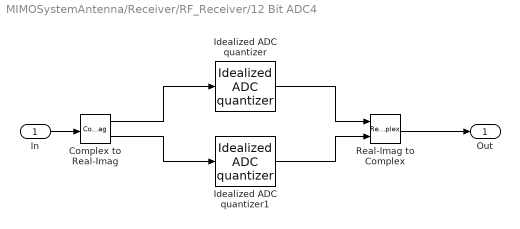
== system MIMOSystemAntenna/Receiver/RF_Receiver/12 Bit ADC4 ==
  "In  " : Inport
  Complex to Real-Imag : ComplexToRealImag
  Idealized ADC quantizer : simulink_extras/Additional Discrete/Idealized ADC quantizer  NumberOfConverterBits=N  Vmin=-10^((FS_P_dBm-30)/20)  Vmax=10^((FS_P_dBm-30)/20)  OutputDataType=double  OutputNegativeValues=on
  Idealized ADC quantizer1 : simulink_extras/Additional Discrete/Idealized ADC quantizer  NumberOfConverterBits=N  Vmin=-10^((FS_P_dBm-30)/20)  Vmax=10^((FS_P_dBm-30)/20)  OutputDataType=double  OutputNegativeValues=on
  Real-Imag to Complex : RealImagToComplex
  Out : Outport  VectorParamsAs1DForOutWhenUnconnected=off
  wires:
  Real-Imag to Complex/1 -> Out/1
  Idealized ADC quantizer1/1 -> Real-Imag to Complex/2
  Idealized ADC quantizer/1 -> Real-Imag to Complex/1
  Complex to Real-Imag/2 -> Idealized ADC quantizer1/1
  Complex to Real-Imag/1 -> Idealized ADC quantizer/1
  "In  "/1 -> Complex to Real-Imag/1

== system MIMOSystemAntenna/Receiver/RF_Receiver/12 Bit ADC5 ==
  "In  " : Inport
  Complex to Real-Imag : ComplexToRealImag
  Idealized ADC quantizer : simulink_extras/Additional Discrete/Idealized ADC quantizer  NumberOfConverterBits=N  Vmin=-10^((FS_P_dBm-30)/20)  Vmax=10^((FS_P_dBm-30)/20)  OutputDataType=double  OutputNegativeValues=on
  Idealized ADC quantizer1 : simulink_extras/Additional Discrete/Idealized ADC quantizer  NumberOfConverterBits=N  Vmin=-10^((FS_P_dBm-30)/20)  Vmax=10^((FS_P_dBm-30)/20)  OutputDataType=double  OutputNegativeValues=on
  Real-Imag to Complex : RealImagToComplex
  Out : Outport  VectorParamsAs1DForOutWhenUnconnected=off
  wires:
  "In  "/1 -> Complex to Real-Imag/1
  Complex to Real-Imag/1 -> Idealized ADC quantizer/1
  Complex to Real-Imag/2 -> Idealized ADC quantizer1/1
  Idealized ADC quantizer/1 -> Real-Imag to Complex/1
  Idealized ADC quantizer1/1 -> Real-Imag to Complex/2
  Real-Imag to Complex/1 -> Out/1

== system MIMOSystemAntenna/Receiver/RF_Receiver/12 Bit ADC6 ==
  "In  " : Inport
  Complex to Real-Imag : ComplexToRealImag
  Idealized ADC quantizer : simulink_extras/Additional Discrete/Idealized ADC quantizer  NumberOfConverterBits=N  Vmin=-10^((FS_P_dBm-30)/20)  Vmax=10^((FS_P_dBm-30)/20)  OutputDataType=double  OutputNegativeValues=on
  Idealized ADC quantizer1 : simulink_extras/Additional Discrete/Idealized ADC quantizer  NumberOfConverterBits=N  Vmin=-10^((FS_P_dBm-30)/20)  Vmax=10^((FS_P_dBm-30)/20)  OutputDataType=double  OutputNegativeValues=on
  Real-Imag to Complex : RealImagToComplex
  Out : Outport  VectorParamsAs1DForOutWhenUnconnected=off
  wires:
  Real-Imag to Complex/1 -> Out/1
  Idealized ADC quantizer1/1 -> Real-Imag to Complex/2
  Idealized ADC quantizer/1 -> Real-Imag to Complex/1
  Complex to Real-Imag/2 -> Idealized ADC quantizer1/1
  Complex to Real-Imag/1 -> Idealized ADC quantizer/1
  "In  "/1 -> Complex to Real-Imag/1

== system MIMOSystemAntenna/Receiver/RF_Receiver/12 Bit ADC7 ==
  "In  " : Inport
  Complex to Real-Imag : ComplexToRealImag
  Idealized ADC quantizer : simulink_extras/Additional Discrete/Idealized ADC quantizer  NumberOfConverterBits=N  Vmin=-10^((FS_P_dBm-30)/20)  Vmax=10^((FS_P_dBm-30)/20)  OutputDataType=double  OutputNegativeValues=on
  Idealized ADC quantizer1 : simulink_extras/Additional Discrete/Idealized ADC quantizer  NumberOfConverterBits=N  Vmin=-10^((FS_P_dBm-30)/20)  Vmax=10^((FS_P_dBm-30)/20)  OutputDataType=double  OutputNegativeValues=on
  Real-Imag to Complex : RealImagToComplex
  Out : Outport  VectorParamsAs1DForOutWhenUnconnected=off
  wires:
  "In  "/1 -> Complex to Real-Imag/1
  Complex to Real-Imag/1 -> Idealized ADC quantizer/1
  Complex to Real-Imag/2 -> Idealized ADC quantizer1/1
  Idealized ADC quantizer/1 -> Real-Imag to Complex/1
  Idealized ADC quantizer1/1 -> Real-Imag to Complex/2
  Real-Imag to Complex/1 -> Out/1

== system MIMOSystemAntenna/Receiver/RF_Receiver/12 Bit ADC8 ==
  "In  " : Inport
  Complex to Real-Imag : ComplexToRealImag
  Idealized ADC quantizer : simulink_extras/Additional Discrete/Idealized ADC quantizer  NumberOfConverterBits=N  Vmin=-10^((FS_P_dBm-30)/20)  Vmax=10^((FS_P_dBm-30)/20)  OutputDataType=double  OutputNegativeValues=on
  Idealized ADC quantizer1 : simulink_extras/Additional Discrete/Idealized ADC quantizer  NumberOfConverterBits=N  Vmin=-10^((FS_P_dBm-30)/20)  Vmax=10^((FS_P_dBm-30)/20)  OutputDataType=double  OutputNegativeValues=on
  Real-Imag to Complex : RealImagToComplex
  Out : Outport  VectorParamsAs1DForOutWhenUnconnected=off
  wires:
  Real-Imag to Complex/1 -> Out/1
  Idealized ADC quantizer1/1 -> Real-Imag to Complex/2
  Idealized ADC quantizer/1 -> Real-Imag to Complex/1
  Complex to Real-Imag/2 -> Idealized ADC quantizer1/1
  Complex to Real-Imag/1 -> Idealized ADC quantizer/1
  "In  "/1 -> Complex to Real-Imag/1

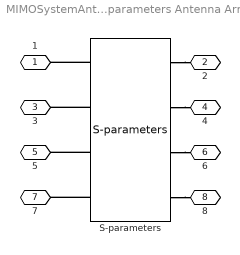
== system MIMOSystemAntenna/Receiver/RF_Receiver/S_parameters Antenna Array ==
  S-parameters : simrfV2elements/S-parameters  classname=sparam_element  DataSource=Network-parameters  File=unitygain.s2p  Paramtype=S-parameters  Sparam=s.Parameters  SparamFreq=s.Frequencies Hz  SparamZ0=50  Residues=0  Poles=0  DF={0 0; 1 0}  FitOpt=Share all poles  FitTol=-40  SourceFreq=Extracted from data source  PlotFreq=[1e9:1e6:3e9] Hz  PlotType=X-Y plane  YParam1=S(1,1)  YFormat1=Magnitude (decibels)  YParam2=None  YFormat2=Magnitude (decibels)  YOption=Linear  XOption=Linear  AddNoise=on  InternalGrounding=on  SparamRepresentation=Frequency domain  AutoImpulseLength=on  ImpulseLength=1e-10 s  MagModeling=off  CacheLevel=0
      settings: SourceProductBaseCode=RB
  1 : PMIOPort  Side=Right
  2 : PMIOPort  Port=2  Side=Right
  3 : PMIOPort  Port=3  Side=Right
  4 : PMIOPort  Port=4  Side=Right
  5 : PMIOPort  Port=5  Side=Right
  6 : PMIOPort  Port=6  Side=Right
  7 : PMIOPort  Port=7  Side=Right
  8 : PMIOPort  Port=8  Side=Right
  connections:
  S-parameters/RConn1 -- 2/RConn1
  S-parameters/LConn4 -- 7/RConn1
  S-parameters/LConn3 -- 5/RConn1
  S-parameters/RConn3 -- 6/RConn1
  S-parameters/LConn2 -- 3/RConn1
  S-parameters/RConn4 -- 8/RConn1
  S-parameters/RConn2 -- 4/RConn1
  S-parameters/LConn1 -- 1/RConn1

== stateflow chart MIMOSystemAntenna/Control Logic/Chart ==
  settings: updateMethod=DISCRETE  sampleTime=8.6806e-08*Frame
  state Steady_State
  state First_Angle
    entry:  Angle= [Directions(1);0];
  state Second_Angle
    entry:  Angle= [Directions(2);0];
  (default) -> Steady_State : {Angle=[0;0];}
  Second_Angle -> Steady_State [order 1] : [after (5, tick) && MER>5]
  Steady_State -> First_Angle : [after(5, tick) && MER<5]
  First_Angle -> Steady_State [order 2] : [after (5, tick) && MER>5]
  Second_Angle -> Second_Angle [order 3] : after(5,tick)
  First_Angle -> First_Angle [order 3] : after(5,tick)
  Second_Angle -> First_Angle [order 2] : [after (5, tick) && MER<0]
  First_Angle -> Second_Angle [order 1] : [after (5, tick) && MER<0]
  data: MER input; Directions input; Angle output double size=[2 1]
